simulink model "SingleTrackCANoe"  (R2021b)
settings: Solver=ode1  StartTime=0  StopTime=2  FixedStep=1.0000000000000000e-003  RelTol=1e-3
InitFcn:
  | sampleTime = str2double(get_param(bdroot, 'FixedStep'));
undefined symbols (not defined in the file or in its folder): AccPedalPos, BrakePedalPos, BrakeSwitch, DiscIntNeverNeededParam, DYNA4, EngSpd, IgnitionSwitch, InitialGear, InitialSpeed, IntendedEngTrq, LeftIndicator, MainBrakePress, MaxGear, MDL, MinGear, RefAcc, RefLane, RefLatPos, RefPath, RefPathCurv, RefSpd, RefSpdPreview, RefSpdRetrospect, RightIndicator, SteeringWheelAng, SteeringWheelTrq, UserDefinedRefValue, vm_const
libraries: UtilitiesLibrary x62, simulink x18, WheelSystemModules x14, LongitudinalControllerModules x13, LateralControllerModules x7, AnimationBusselectorModules x5, EnvironmentModules x5, BasicEngineControlModules x5, MiscellaneousControlModules x5, Animation3Modules x4, AuxiliariesModules x4, ReducedTireModules x4
(part 32 of 34)

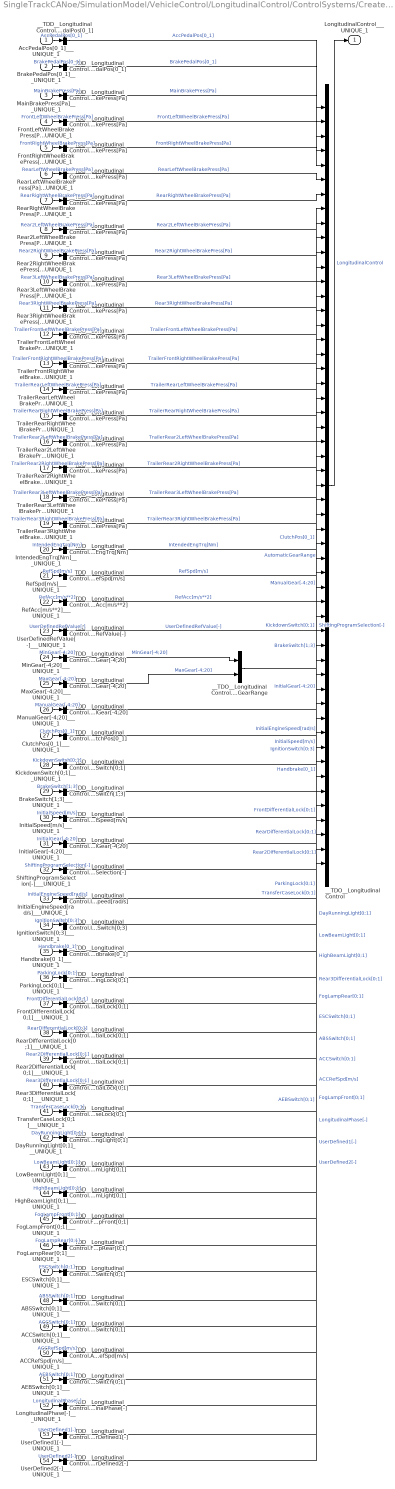
== system SingleTrackCANoe/SimulationModel/VehicleControl/LongitudinalControl/ControlSystems/CreateOutputBus/LongitudinalControlOutput ==
  AccPedalPos[0_1]___UNIQUE_1 : Inport  Description=|  PortDimensions=[1]
      | <name>AccPedalPos[0_1]</name>
      | <comment>Accelerator pedal position</comment>
  BrakePedalPos[0_1]___UNIQUE_1 : Inport  Description=|  Port=2  PortDimensions=[1]
      | <name>BrakePedalPos[0_1]</name>
      | <comment>Brake pedal position</comment>
  MainBrakePress[Pa]___UNIQUE_1 : Inport  Description=|  Port=3  PortDimensions=[1]
      | <name>MainBrakePress[Pa]</name>
      | <comment>Main brake pressure</comment>
  FrontLeftWheelBrakePress[Pa]___UNIQUE_1 : Inport  Description=|  Port=4  PortDimensions=[1]
      | <name>FrontLeftWheelBrakePress[Pa]</name>
      | <comment>Front axle left wheel brake pressure</comment>
  FrontRightWheelBrakePress[Pa]___UNIQUE_1 : Inport  Description=|  Port=5  PortDimensions=[1]
      | <name>FrontRightWheelBrakePress[Pa]</name>
      | <comment>Front axle right wheel brake pressure</comment>
  RearLeftWheelBrakePress[Pa]___UNIQUE_1 : Inport  Description=|  Port=6  PortDimensions=[1]
      | <name>RearLeftWheelBrakePress[Pa]</name>
      | <comment>Rear axle left wheel brake pressure</comment>
  RearRightWheelBrakePress[Pa]___UNIQUE_1 : Inport  Description=|  Port=7  PortDimensions=[1]
      | <name>RearRightWheelBrakePress[Pa]</name>
      | <comment>Rear axle right wheel brake pressure</comment>
  Rear2LeftWheelBrakePress[Pa]___UNIQUE_1 : Inport  Description=|  Port=8  PortDimensions=[1]
      | <name>Rear2LeftWheelBrakePress[Pa]</name>
      | <comment>Second rear axle left wheel brake pressure</comment>
  Rear2RightWheelBrakePress[Pa]___UNIQUE_1 : Inport  Description=|  Port=9  PortDimensions=[1]
      | <name>Rear2RightWheelBrakePress[Pa]</name>
      | <comment>Second rear axle right wheel brake pressure</comment>
  Rear3LeftWheelBrakePress[Pa]___UNIQUE_1 : Inport  Description=|  Port=10  PortDimensions=[1]
      | <name>Rear3LeftWheelBrakePress[Pa]</name>
      | <comment>Third rear axle left wheel brake pressure</comment>
  Rear3RightWheelBrakePress[Pa]___UNIQUE_1 : Inport  Description=|  Port=11  PortDimensions=[1]
      | <name>Rear3RightWheelBrakePress[Pa]</name>
      | <comment>Third rear axle right wheel brake pressure</comment>
  TrailerFrontLeftWheelBrakePress[Pa]___UNIQUE_1 : Inport  Description=|  Port=12  PortDimensions=[1]
      | <name>TrailerFrontLeftWheelBrakePress[Pa]</name>
      | <comment>Trailer front axle left wheel brake pressure</comment>
  TrailerFrontRightWheelBrakePress[Pa]___UNIQUE_1 : Inport  Description=|  Port=13  PortDimensions=[1]
      | <name>TrailerFrontRightWheelBrakePress[Pa]</name>
      | <comment>Trailer front axle right wheel brake pressure</comment>
  TrailerRearLeftWheelBrakePress[Pa]___UNIQUE_1 : Inport  Description=|  Port=14  PortDimensions=[1]
      | <name>TrailerRearLeftWheelBrakePress[Pa]</name>
      | <comment>Trailer rear axle left wheel brake pressure</comment>
  TrailerRearRightWheelBrakePress[Pa]___UNIQUE_1 : Inport  Description=|  Port=15  PortDimensions=[1]
      | <name>TrailerRearRightWheelBrakePress[Pa]</name>
      | <comment>Trailer rear axle right wheel brake pressure</comment>
  TrailerRear2LeftWheelBrakePress[Pa]___UNIQUE_1 : Inport  Description=|  Port=16  PortDimensions=[1]
      | <name>TrailerRear2LeftWheelBrakePress[Pa]</name>
      | <comment>Trailer second rear axle left wheel brake pressure</comment>
  TrailerRear2RightWheelBrakePress[Pa]___UNIQUE_1 : Inport  Description=|  Port=17  PortDimensions=[1]
      | <name>TrailerRear2RightWheelBrakePress[Pa]</name>
      | <comment>Trailer second rear axle right wheel brake pressure</comment>
  TrailerRear3LeftWheelBrakePress[Pa]___UNIQUE_1 : Inport  Description=|  Port=18  PortDimensions=[1]
      | <name>TrailerRear3LeftWheelBrakePress[Pa]</name>
      | <comment>Trailer third rear axle left wheel brake pressure</comment>
  TrailerRear3RightWheelBrakePress[Pa]___UNIQUE_1 : Inport  Description=|  Port=19  PortDimensions=[1]
      | <name>TrailerRear3RightWheelBrakePress[Pa]</name>
      | <comment>Trailer third rear axle right wheel brake pressure</comment>
  IntendedEngTrq[Nm]___UNIQUE_1 : Inport  Description=|  Port=20  PortDimensions=[1]
      | <name>IntendedEngTrq[Nm]</name>
      | <comment>Intended engine torque</comment>
  RefSpd[m/s]___UNIQUE_1 : Inport  Description=|  Port=21  PortDimensions=[1]
      | <name>RefSpd[m/s]</name>
      | <comment>Vehicle reference speed</comment>
  RefAcc[m/s**2]___UNIQUE_1 : Inport  Description=|  Port=22  PortDimensions=[1]
      | <name>RefAcc[m/s**2]</name>
      | <comment></comment>
  UserDefinedRefValue[-]___UNIQUE_1 : Inport  Description=|  Port=23  PortDimensions=[1]
      | <name>UserDefinedRefValue[-]</name>
      | <comment>User-defined reference value</comment>
  MinGear[-4;20]___UNIQUE_1 : Inport  Description=|  Port=24  PortDimensions=[1]
      | <name>MinGear[-4;20]</name>
      | <comment>Minimum gear</comment>
  MaxGear[-4;20]___UNIQUE_1 : Inport  Description=|  Port=25  PortDimensions=[1]
      | <name>MaxGear[-4;20]</name>
      | <comment>Maximum gear</comment>
  ManualGear[-4;20]___UNIQUE_1 : Inport  Description=|  Port=26  PortDimensions=[1]
      | <name>ManualGear[-4;20]</name>
      | <comment>Gear number for manual transmission</comment>
  ClutchPos[0_1]___UNIQUE_1 : Inport  Description=|  Port=27  PortDimensions=[1]
      | <name>ClutchPos[0_1]</name>
      | <comment>Clutch position</comment>
  KickdownSwitch[0;1]___UNIQUE_1 : Inport  Description=|  Port=28  PortDimensions=[1]
      | <name>KickdownSwitch[0;1]</name>
      | <comment>Kickdown switch</comment>
  BrakeSwitch[1;3]___UNIQUE_1 : Inport  Description=|  Port=29  PortDimensions=[1]
      | <name>BrakeSwitch[1;3]</name>
      | <comment>Logical switch for brake system control, 1: Main and wheel brake pressures are calculated from the supplied brake pedal position, 2: Wheel brake pressures are calculated from the supplied main brake pressure, 3: Wheel brake pressures are supplied directly </comment>
  InitialSpeed[m/s]___UNIQUE_1 : Inport  Description=|  Port=30  PortDimensions=[1]
      | <name>InitialSpeed[m/s]</name>
      | <comment>Initial vehicle speed</comment>
  InitialGear[-4;20]___UNIQUE_1 : Inport  Description=|  Port=31  PortDimensions=[1]
      | <name>InitialGear[-4;20]</name>
      | <comment>Initial gear</comment>
  ShiftingProgramSelection[-]___UNIQUE_1 : Inport  Description=|  Port=32  PortDimensions=[1]
      | <name>ShiftingProgramSelection[-]</name>
      | <comment>Selection of shifting program number</comment>
  InitialEngineSpeed[rad/s]___UNIQUE_1 : Inport  Description=|  Port=33  PortDimensions=[1]
      | <name>InitialEngineSpeed[rad/s]</name>
      | <comment>Initial engine speed</comment>
  IgnitionSwitch[0;3]___UNIQUE_1 : Inport  Description=|  Port=34  PortDimensions=[1]
      | <name>IgnitionSwitch[0;3]</name>
      | <comment>Ignition switch, 0: Ignition is off,  1: Only limited electric power supply, e.g for the radio, is available, 2: Normal operation mode: Full electric power supply is available, 3: Starter is activated</comment>
  Handbrake[0_1]___UNIQUE_1 : Inport  Description=|  Port=35  PortDimensions=[1]
      | <name>Handbrake[0_1]</name>
      | <comment>Handbrake position</comment>
  ParkingLock[0;1]___UNIQUE_1 : Inport  Description=|  Port=36  PortDimensions=[1]
      | <name>ParkingLock[0;1]</name>
      | <comment>Parking lock state</comment>
  FrontDifferentialLock[0;1]___UNIQUE_1 : Inport  Description=|  Port=37  PortDimensions=[1]
      | <name>FrontDifferentialLock[0;1]</name>
      | <comment>Front differential lock state</comment>
  RearDifferentialLock[0;1]___UNIQUE_1 : Inport  Description=|  Port=38  PortDimensions=[1]
      | <name>RearDifferentialLock[0;1]</name>
      | <comment>Rear differential lock state</comment>
  Rear2DifferentialLock[0;1]___UNIQUE_1 : Inport  Description=|  Port=39  PortDimensions=[1]
      | <name>Rear2DifferentialLock[0;1]</name>
      | <comment>Second rear differential lock state</comment>
  Rear3DifferentialLock[0;1]___UNIQUE_1 : Inport  Description=|  Port=40  PortDimensions=[1]
      | <name>Rear3DifferentialLock[0;1]</name>
      | <comment>Third rear differential lock state</comment>
  TransferCaseLock[0;1]___UNIQUE_1 : Inport  Description=|  Port=41  PortDimensions=[1]
      | <name>TransferCaseLock[0;1]</name>
      | <comment>Transfer case lock state</comment>
  DayRunningLight[0;1]___UNIQUE_1 : Inport  Description=|  Port=42  PortDimensions=[1]
      | <name>DayRunningLight[0;1]</name>
      | <comment></comment>
  LowBeamLight[0;1]___UNIQUE_1 : Inport  Description=|  Port=43  PortDimensions=[1]
      | <name>LowBeamLight[0;1]</name>
      | <comment></comment>
  HighBeamLight[0;1]___UNIQUE_1 : Inport  Description=|  Port=44  PortDimensions=[1]
      | <name>HighBeamLight[0;1]</name>
      | <comment></comment>
  FogLampFront[0;1]___UNIQUE_1 : Inport  Description=|  Port=45  PortDimensions=[1]
      | <name>FogLampFront[0;1]</name>
      | <comment></comment>
  FogLampRear[0;1]___UNIQUE_1 : Inport  Description=|  Port=46  PortDimensions=[1]
      | <name>FogLampRear[0;1]</name>
      | <comment></comment>
  ESCSwitch[0;1]___UNIQUE_1 : Inport  Description=|  Port=47  PortDimensions=[1]
      | <name>ESCSwitch[0;1]</name>
      | <comment>ESC activation switch</comment>
  ABSSwitch[0;1]___UNIQUE_1 : Inport  Description=|  Port=48  PortDimensions=[1]
      | <name>ABSSwitch[0;1]</name>
      | <comment>ABS activation switch</comment>
  ACCSwitch[0;1]___UNIQUE_1 : Inport  Description=|  Port=49  PortDimensions=[1]
      | <name>ACCSwitch[0;1]</name>
      | <comment></comment>
  ACCRefSpd[m/s]___UNIQUE_1 : Inport  Description=|  Port=50  PortDimensions=[1]
      | <name>ACCRefSpd[m/s]</name>
      | <comment></comment>
  AEBSwitch[0;1]___UNIQUE_1 : Inport  Description=|  Port=51  PortDimensions=[1]
      | <name>AEBSwitch[0;1]</name>
      | <comment></comment>
  LongitudinalPhase[-]___UNIQUE_1 : Inport  Description=|  Port=52  PortDimensions=[1]
      | <name>LongitudinalPhase[-]</name>
      | <comment>Longitudinal phase number</comment>
  UserDefined1[-]___UNIQUE_1 : Inport  Description=|  Port=53  PortDimensions=[1]
      | <name>UserDefined.UserDefined1[-]</name>
      | <comment>User-defined additional input 1 (can be edited by the user)</comment>
  UserDefined2[-]___UNIQUE_1 : Inport  Description=|  Port=54  PortDimensions=[1]
      | <name>UserDefined.UserDefined2[-]</name>
      | <comment>User-defined additional input 2 (can be edited by the user)</comment>
  __TDD__LongitudinalControl.ABSSwitch[0;1] : Demux  Outputs=[1]
  __TDD__LongitudinalControl.ACCRefSpd[m/s] : Demux  Outputs=[1]
  __TDD__LongitudinalControl.ACCSwitch[0;1] : Demux  Outputs=[1]
  __TDD__LongitudinalControl.AEBSwitch[0;1] : Demux  Outputs=[1]
  __TDD__LongitudinalControl.AccPedalPos[0_1] : Demux  Outputs=[1]
  __TDD__LongitudinalControl.AutomaticGearRange.MaxGear[-4;20] : Demux  Outputs=[1]
  __TDD__LongitudinalControl.AutomaticGearRange.MinGear[-4;20] : Demux  Outputs=[1]
  __TDD__LongitudinalControl.BrakePedalPos[0_1] : Demux  Outputs=[1]
  __TDD__LongitudinalControl.BrakeSwitch[1;3] : Demux  Outputs=[1]
  __TDD__LongitudinalControl.ClutchPos[0_1] : Demux  Outputs=[1]
  __TDD__LongitudinalControl.DayRunningLight[0;1] : Demux  Outputs=[1]
  __TDD__LongitudinalControl.ESCSwitch[0;1] : Demux  Outputs=[1]
  __TDD__LongitudinalControl.FogLampFront[0;1] : Demux  Outputs=[1]
  __TDD__LongitudinalControl.FogLampRear[0;1] : Demux  Outputs=[1]
  __TDD__LongitudinalControl.FrontDifferentialLock[0;1] : Demux  Outputs=[1]
  __TDD__LongitudinalControl.FrontLeftWheelBrakePress[Pa] : Demux  Outputs=[1]
  __TDD__LongitudinalControl.FrontRightWheelBrakePress[Pa] : Demux  Outputs=[1]
  __TDD__LongitudinalControl.Handbrake[0_1] : Demux  Outputs=[1]
  __TDD__LongitudinalControl.HighBeamLight[0;1] : Demux  Outputs=[1]
  __TDD__LongitudinalControl.IgnitionSwitch[0;3] : Demux  Outputs=[1]
  __TDD__LongitudinalControl.InitialEngineSpeed[rad/s] : Demux  Outputs=[1]
  __TDD__LongitudinalControl.InitialGear[-4;20] : Demux  Outputs=[1]
  __TDD__LongitudinalControl.InitialSpeed[m/s] : Demux  Outputs=[1]
  __TDD__LongitudinalControl.IntendedEngTrq[Nm] : Demux  Outputs=[1]
  __TDD__LongitudinalControl.KickdownSwitch[0;1] : Demux  Outputs=[1]
  __TDD__LongitudinalControl.LongitudinalPhase[-] : Demux  Outputs=[1]
  __TDD__LongitudinalControl.LowBeamLight[0;1] : Demux  Outputs=[1]
  __TDD__LongitudinalControl.MainBrakePress[Pa] : Demux  Outputs=[1]
  __TDD__LongitudinalControl.ManualGear[-4;20] : Demux  Outputs=[1]
  __TDD__LongitudinalControl.ParkingLock[0;1] : Demux  Outputs=[1]
  __TDD__LongitudinalControl.Rear2DifferentialLock[0;1] : Demux  Outputs=[1]
  __TDD__LongitudinalControl.Rear2LeftWheelBrakePress[Pa] : Demux  Outputs=[1]
  __TDD__LongitudinalControl.Rear2RightWheelBrakePress[Pa] : Demux  Outputs=[1]
  __TDD__LongitudinalControl.Rear3DifferentialLock[0;1] : Demux  Outputs=[1]
  __TDD__LongitudinalControl.Rear3LeftWheelBrakePress[Pa] : Demux  Outputs=[1]
  __TDD__LongitudinalControl.Rear3RightWheelBrakePress[Pa] : Demux  Outputs=[1]
  __TDD__LongitudinalControl.RearDifferentialLock[0;1] : Demux  Outputs=[1]
  __TDD__LongitudinalControl.RearLeftWheelBrakePress[Pa] : Demux  Outputs=[1]
  __TDD__LongitudinalControl.RearRightWheelBrakePress[Pa] : Demux  Outputs=[1]
  __TDD__LongitudinalControl.RefAcc[m/s**2] : Demux  Outputs=[1]
  __TDD__LongitudinalControl.RefSpd[m/s] : Demux  Outputs=[1]
  __TDD__LongitudinalControl.ShiftingProgramSelection[-] : Demux  Outputs=[1]
  __TDD__LongitudinalControl.TrailerFrontLeftWheelBrakePress[Pa] : Demux  Outputs=[1]
  __TDD__LongitudinalControl.TrailerFrontRightWheelBrakePress[Pa] : Demux  Outputs=[1]
  __TDD__LongitudinalControl.TrailerRear2LeftWheelBrakePress[Pa] : Demux  Outputs=[1]
  __TDD__LongitudinalControl.TrailerRear2RightWheelBrakePress[Pa] : Demux  Outputs=[1]
  __TDD__LongitudinalControl.TrailerRear3LeftWheelBrakePress[Pa] : Demux  Outputs=[1]
  __TDD__LongitudinalControl.TrailerRear3RightWheelBrakePress[Pa] : Demux  Outputs=[1]
  __TDD__LongitudinalControl.TrailerRearLeftWheelBrakePress[Pa] : Demux  Outputs=[1]
  __TDD__LongitudinalControl.TrailerRearRightWheelBrakePress[Pa] : Demux  Outputs=[1]
  __TDD__LongitudinalControl.TransferCaseLock[0;1] : Demux  Outputs=[1]
  __TDD__LongitudinalControl.UserDefined1[-] : Demux  Outputs=[1]
  __TDD__LongitudinalControl.UserDefined2[-] : Demux  Outputs=[1]
  __TDD__LongitudinalControl.UserDefinedRefValue[-] : Demux  Outputs=[1]
  __TDO__LongitudinalControl : BusCreator  Inputs=53
  __TDO__LongitudinalControl.AutomaticGearRange : BusCreator  Inputs=2
  LongitudinalControl___UNIQUE_1 : Outport  Description=|  PortDimensions=[54]  VectorParamsAs1DForOutWhenUnconnected=off
      | <name>AccPedalPos[0_1]</name>
      | <comment>Accelerator pedal position</comment>
  wires:
  AccPedalPos[0_1]___UNIQUE_1/1 -> __TDD__LongitudinalControl.AccPedalPos[0_1]/1  "AccPedalPos[0_1]"
  __TDD__LongitudinalControl.AccPedalPos[0_1]/1 -> __TDO__LongitudinalControl/1  "AccPedalPos[0_1]"
  BrakePedalPos[0_1]___UNIQUE_1/1 -> __TDD__LongitudinalControl.BrakePedalPos[0_1]/1  "BrakePedalPos[0_1]"
  __TDD__LongitudinalControl.BrakePedalPos[0_1]/1 -> __TDO__LongitudinalControl/2  "BrakePedalPos[0_1]"
  MainBrakePress[Pa]___UNIQUE_1/1 -> __TDD__LongitudinalControl.MainBrakePress[Pa]/1  "MainBrakePress[Pa]"
  __TDD__LongitudinalControl.MainBrakePress[Pa]/1 -> __TDO__LongitudinalControl/3  "MainBrakePress[Pa]"
  FrontLeftWheelBrakePress[Pa]___UNIQUE_1/1 -> __TDD__LongitudinalControl.FrontLeftWheelBrakePress[Pa]/1  "FrontLeftWheelBrakePress[Pa]"
  __TDD__LongitudinalControl.FrontLeftWheelBrakePress[Pa]/1 -> __TDO__LongitudinalControl/4  "FrontLeftWheelBrakePress[Pa]"
  FrontRightWheelBrakePress[Pa]___UNIQUE_1/1 -> __TDD__LongitudinalControl.FrontRightWheelBrakePress[Pa]/1  "FrontRightWheelBrakePress[Pa]"
  __TDD__LongitudinalControl.FrontRightWheelBrakePress[Pa]/1 -> __TDO__LongitudinalControl/5  "FrontRightWheelBrakePress[Pa]"
  RearLeftWheelBrakePress[Pa]___UNIQUE_1/1 -> __TDD__LongitudinalControl.RearLeftWheelBrakePress[Pa]/1  "RearLeftWheelBrakePress[Pa]"
  __TDD__LongitudinalControl.RearLeftWheelBrakePress[Pa]/1 -> __TDO__LongitudinalControl/6  "RearLeftWheelBrakePress[Pa]"
  RearRightWheelBrakePress[Pa]___UNIQUE_1/1 -> __TDD__LongitudinalControl.RearRightWheelBrakePress[Pa]/1  "RearRightWheelBrakePress[Pa]"
  __TDD__LongitudinalControl.RearRightWheelBrakePress[Pa]/1 -> __TDO__LongitudinalControl/7  "RearRightWheelBrakePress[Pa]"
  Rear2LeftWheelBrakePress[Pa]___UNIQUE_1/1 -> __TDD__LongitudinalControl.Rear2LeftWheelBrakePress[Pa]/1  "Rear2LeftWheelBrakePress[Pa]"
  __TDD__LongitudinalControl.Rear2LeftWheelBrakePress[Pa]/1 -> __TDO__LongitudinalControl/8  "Rear2LeftWheelBrakePress[Pa]"
  Rear2RightWheelBrakePress[Pa]___UNIQUE_1/1 -> __TDD__LongitudinalControl.Rear2RightWheelBrakePress[Pa]/1  "Rear2RightWheelBrakePress[Pa]"
  __TDD__LongitudinalControl.Rear2RightWheelBrakePress[Pa]/1 -> __TDO__LongitudinalControl/9  "Rear2RightWheelBrakePress[Pa]"
  Rear3LeftWheelBrakePress[Pa]___UNIQUE_1/1 -> __TDD__LongitudinalControl.Rear3LeftWheelBrakePress[Pa]/1  "Rear3LeftWheelBrakePress[Pa]"
  __TDD__LongitudinalControl.Rear3LeftWheelBrakePress[Pa]/1 -> __TDO__LongitudinalControl/10  "Rear3LeftWheelBrakePress[Pa]"
  Rear3RightWheelBrakePress[Pa]___UNIQUE_1/1 -> __TDD__LongitudinalControl.Rear3RightWheelBrakePress[Pa]/1  "Rear3RightWheelBrakePress[Pa]"
  __TDD__LongitudinalControl.Rear3RightWheelBrakePress[Pa]/1 -> __TDO__LongitudinalControl/11  "Rear3RightWheelBrakePress[Pa]"
  TrailerFrontLeftWheelBrakePress[Pa]___UNIQUE_1/1 -> __TDD__LongitudinalControl.TrailerFrontLeftWheelBrakePress[Pa]/1  "TrailerFrontLeftWheelBrakePress[Pa]"
  __TDD__LongitudinalControl.TrailerFrontLeftWheelBrakePress[Pa]/1 -> __TDO__LongitudinalControl/12  "TrailerFrontLeftWheelBrakePress[Pa]"
  TrailerFrontRightWheelBrakePress[Pa]___UNIQUE_1/1 -> __TDD__LongitudinalControl.TrailerFrontRightWheelBrakePress[Pa]/1  "TrailerFrontRightWheelBrakePress[Pa]"
  __TDD__LongitudinalControl.TrailerFrontRightWheelBrakePress[Pa]/1 -> __TDO__LongitudinalControl/13  "TrailerFrontRightWheelBrakePress[Pa]"
  TrailerRearLeftWheelBrakePress[Pa]___UNIQUE_1/1 -> __TDD__LongitudinalControl.TrailerRearLeftWheelBrakePress[Pa]/1  "TrailerRearLeftWheelBrakePress[Pa]"
  __TDD__LongitudinalControl.TrailerRearLeftWheelBrakePress[Pa]/1 -> __TDO__LongitudinalControl/14  "TrailerRearLeftWheelBrakePress[Pa]"
  TrailerRearRightWheelBrakePress[Pa]___UNIQUE_1/1 -> __TDD__LongitudinalControl.TrailerRearRightWheelBrakePress[Pa]/1  "TrailerRearRightWheelBrakePress[Pa]"
  __TDD__LongitudinalControl.TrailerRearRightWheelBrakePress[Pa]/1 -> __TDO__LongitudinalControl/15  "TrailerRearRightWheelBrakePress[Pa]"
  TrailerRear2LeftWheelBrakePress[Pa]___UNIQUE_1/1 -> __TDD__LongitudinalControl.TrailerRear2LeftWheelBrakePress[Pa]/1  "TrailerRear2LeftWheelBrakePress[Pa]"
  __TDD__LongitudinalControl.TrailerRear2LeftWheelBrakePress[Pa]/1 -> __TDO__LongitudinalControl/16  "TrailerRear2LeftWheelBrakePress[Pa]"
  TrailerRear2RightWheelBrakePress[Pa]___UNIQUE_1/1 -> __TDD__LongitudinalControl.TrailerRear2RightWheelBrakePress[Pa]/1  "TrailerRear2RightWheelBrakePress[Pa]"
  __TDD__LongitudinalControl.TrailerRear2RightWheelBrakePress[Pa]/1 -> __TDO__LongitudinalControl/17  "TrailerRear2RightWheelBrakePress[Pa]"
  TrailerRear3LeftWheelBrakePress[Pa]___UNIQUE_1/1 -> __TDD__LongitudinalControl.TrailerRear3LeftWheelBrakePress[Pa]/1  "TrailerRear3LeftWheelBrakePress[Pa]"
  __TDD__LongitudinalControl.TrailerRear3LeftWheelBrakePress[Pa]/1 -> __TDO__LongitudinalControl/18  "TrailerRear3LeftWheelBrakePress[Pa]"
  TrailerRear3RightWheelBrakePress[Pa]___UNIQUE_1/1 -> __TDD__LongitudinalControl.TrailerRear3RightWheelBrakePress[Pa]/1  "TrailerRear3RightWheelBrakePress[Pa]"
  __TDD__LongitudinalControl.TrailerRear3RightWheelBrakePress[Pa]/1 -> __TDO__LongitudinalControl/19  "TrailerRear3RightWheelBrakePress[Pa]"
  IntendedEngTrq[Nm]___UNIQUE_1/1 -> __TDD__LongitudinalControl.IntendedEngTrq[Nm]/1  "IntendedEngTrq[Nm]"
  __TDD__LongitudinalControl.IntendedEngTrq[Nm]/1 -> __TDO__LongitudinalControl/20  "IntendedEngTrq[Nm]"
  RefSpd[m/s]___UNIQUE_1/1 -> __TDD__LongitudinalControl.RefSpd[m/s]/1  "RefSpd[m/s]"
  __TDD__LongitudinalControl.RefSpd[m/s]/1 -> __TDO__LongitudinalControl/21  "RefSpd[m/s]"
  RefAcc[m/s**2]___UNIQUE_1/1 -> __TDD__LongitudinalControl.RefAcc[m/s**2]/1  "RefAcc[m/s**2]"
  __TDD__LongitudinalControl.RefAcc[m/s**2]/1 -> __TDO__LongitudinalControl/22  "RefAcc[m/s**2]"
  UserDefinedRefValue[-]___UNIQUE_1/1 -> __TDD__LongitudinalControl.UserDefinedRefValue[-]/1  "UserDefinedRefValue[-]"
  __TDD__LongitudinalControl.UserDefinedRefValue[-]/1 -> __TDO__LongitudinalControl/23  "UserDefinedRefValue[-]"
  MinGear[-4;20]___UNIQUE_1/1 -> __TDD__LongitudinalControl.AutomaticGearRange.MinGear[-4;20]/1  "MinGear[-4;20]"
  __TDD__LongitudinalControl.AutomaticGearRange.MinGear[-4;20]/1 -> __TDO__LongitudinalControl.AutomaticGearRange/1  "MinGear[-4;20]"
  __TDO__LongitudinalControl.AutomaticGearRange/1 -> __TDO__LongitudinalControl/24  "AutomaticGearRange"
  MaxGear[-4;20]___UNIQUE_1/1 -> __TDD__LongitudinalControl.AutomaticGearRange.MaxGear[-4;20]/1  "MaxGear[-4;20]"
  __TDD__LongitudinalControl.AutomaticGearRange.MaxGear[-4;20]/1 -> __TDO__LongitudinalControl.AutomaticGearRange/2  "MaxGear[-4;20]"
  ManualGear[-4;20]___UNIQUE_1/1 -> __TDD__LongitudinalControl.ManualGear[-4;20]/1  "ManualGear[-4;20]"
  __TDD__LongitudinalControl.ManualGear[-4;20]/1 -> __TDO__LongitudinalControl/25  "ManualGear[-4;20]"
  ClutchPos[0_1]___UNIQUE_1/1 -> __TDD__LongitudinalControl.ClutchPos[0_1]/1  "ClutchPos[0_1]"
  __TDD__LongitudinalControl.ClutchPos[0_1]/1 -> __TDO__LongitudinalControl/26  "ClutchPos[0_1]"
  KickdownSwitch[0;1]___UNIQUE_1/1 -> __TDD__LongitudinalControl.KickdownSwitch[0;1]/1  "KickdownSwitch[0;1]"
  __TDD__LongitudinalControl.KickdownSwitch[0;1]/1 -> __TDO__LongitudinalControl/27  "KickdownSwitch[0;1]"
  BrakeSwitch[1;3]___UNIQUE_1/1 -> __TDD__LongitudinalControl.BrakeSwitch[1;3]/1  "BrakeSwitch[1;3]"
  __TDD__LongitudinalControl.BrakeSwitch[1;3]/1 -> __TDO__LongitudinalControl/28  "BrakeSwitch[1;3]"
  InitialSpeed[m/s]___UNIQUE_1/1 -> __TDD__LongitudinalControl.InitialSpeed[m/s]/1  "InitialSpeed[m/s]"
  __TDD__LongitudinalControl.InitialSpeed[m/s]/1 -> __TDO__LongitudinalControl/29  "InitialSpeed[m/s]"
  InitialGear[-4;20]___UNIQUE_1/1 -> __TDD__LongitudinalControl.InitialGear[-4;20]/1  "InitialGear[-4;20]"
  __TDD__LongitudinalControl.InitialGear[-4;20]/1 -> __TDO__LongitudinalControl/30  "InitialGear[-4;20]"
  ShiftingProgramSelection[-]___UNIQUE_1/1 -> __TDD__LongitudinalControl.ShiftingProgramSelection[-]/1  "ShiftingProgramSelection[-]"
  __TDD__LongitudinalControl.ShiftingProgramSelection[-]/1 -> __TDO__LongitudinalControl/31  "ShiftingProgramSelection[-]"
  InitialEngineSpeed[rad/s]___UNIQUE_1/1 -> __TDD__LongitudinalControl.InitialEngineSpeed[rad/s]/1  "InitialEngineSpeed[rad/s]"
  __TDD__LongitudinalControl.InitialEngineSpeed[rad/s]/1 -> __TDO__LongitudinalControl/32  "InitialEngineSpeed[rad/s]"
  IgnitionSwitch[0;3]___UNIQUE_1/1 -> __TDD__LongitudinalControl.IgnitionSwitch[0;3]/1  "IgnitionSwitch[0;3]"
  __TDD__LongitudinalControl.IgnitionSwitch[0;3]/1 -> __TDO__LongitudinalControl/33  "IgnitionSwitch[0;3]"
  Handbrake[0_1]___UNIQUE_1/1 -> __TDD__LongitudinalControl.Handbrake[0_1]/1  "Handbrake[0_1]"
  __TDD__LongitudinalControl.Handbrake[0_1]/1 -> __TDO__LongitudinalControl/34  "Handbrake[0_1]"
  ParkingLock[0;1]___UNIQUE_1/1 -> __TDD__LongitudinalControl.ParkingLock[0;1]/1  "ParkingLock[0;1]"
  __TDD__LongitudinalControl.ParkingLock[0;1]/1 -> __TDO__LongitudinalControl/35  "ParkingLock[0;1]"
  FrontDifferentialLock[0;1]___UNIQUE_1/1 -> __TDD__LongitudinalControl.FrontDifferentialLock[0;1]/1  "FrontDifferentialLock[0;1]"
  __TDD__LongitudinalControl.FrontDifferentialLock[0;1]/1 -> __TDO__LongitudinalControl/36  "FrontDifferentialLock[0;1]"
  RearDifferentialLock[0;1]___UNIQUE_1/1 -> __TDD__LongitudinalControl.RearDifferentialLock[0;1]/1  "RearDifferentialLock[0;1]"
  __TDD__LongitudinalControl.RearDifferentialLock[0;1]/1 -> __TDO__LongitudinalControl/37  "RearDifferentialLock[0;1]"
  Rear2DifferentialLock[0;1]___UNIQUE_1/1 -> __TDD__LongitudinalControl.Rear2DifferentialLock[0;1]/1  "Rear2DifferentialLock[0;1]"
  __TDD__LongitudinalControl.Rear2DifferentialLock[0;1]/1 -> __TDO__LongitudinalControl/38  "Rear2DifferentialLock[0;1]"
  Rear3DifferentialLock[0;1]___UNIQUE_1/1 -> __TDD__LongitudinalControl.Rear3DifferentialLock[0;1]/1  "Rear3DifferentialLock[0;1]"
  __TDD__LongitudinalControl.Rear3DifferentialLock[0;1]/1 -> __TDO__LongitudinalControl/39  "Rear3DifferentialLock[0;1]"
  TransferCaseLock[0;1]___UNIQUE_1/1 -> __TDD__LongitudinalControl.TransferCaseLock[0;1]/1  "TransferCaseLock[0;1]"
  __TDD__LongitudinalControl.TransferCaseLock[0;1]/1 -> __TDO__LongitudinalControl/40  "TransferCaseLock[0;1]"
  DayRunningLight[0;1]___UNIQUE_1/1 -> __TDD__LongitudinalControl.DayRunningLight[0;1]/1  "DayRunningLight[0;1]"
  __TDD__LongitudinalControl.DayRunningLight[0;1]/1 -> __TDO__LongitudinalControl/41  "DayRunningLight[0;1]"
  LowBeamLight[0;1]___UNIQUE_1/1 -> __TDD__LongitudinalControl.LowBeamLight[0;1]/1  "LowBeamLight[0;1]"
  __TDD__LongitudinalControl.LowBeamLight[0;1]/1 -> __TDO__LongitudinalControl/42  "LowBeamLight[0;1]"
  HighBeamLight[0;1]___UNIQUE_1/1 -> __TDD__LongitudinalControl.HighBeamLight[0;1]/1  "HighBeamLight[0;1]"
  __TDD__LongitudinalControl.HighBeamLight[0;1]/1 -> __TDO__LongitudinalControl/43  "HighBeamLight[0;1]"
  FogLampFront[0;1]___UNIQUE_1/1 -> __TDD__LongitudinalControl.FogLampFront[0;1]/1  "FogLampFront[0;1]"
  __TDD__LongitudinalControl.FogLampFront[0;1]/1 -> __TDO__LongitudinalControl/44  "FogLampFront[0;1]"
  FogLampRear[0;1]___UNIQUE_1/1 -> __TDD__LongitudinalControl.FogLampRear[0;1]/1  "FogLampRear[0;1]"
  __TDD__LongitudinalControl.FogLampRear[0;1]/1 -> __TDO__LongitudinalControl/45  "FogLampRear[0;1]"
  ESCSwitch[0;1]___UNIQUE_1/1 -> __TDD__LongitudinalControl.ESCSwitch[0;1]/1  "ESCSwitch[0;1]"
  __TDD__LongitudinalControl.ESCSwitch[0;1]/1 -> __TDO__LongitudinalControl/46  "ESCSwitch[0;1]"
  ABSSwitch[0;1]___UNIQUE_1/1 -> __TDD__LongitudinalControl.ABSSwitch[0;1]/1  "ABSSwitch[0;1]"
  __TDD__LongitudinalControl.ABSSwitch[0;1]/1 -> __TDO__LongitudinalControl/47  "ABSSwitch[0;1]"
  ACCSwitch[0;1]___UNIQUE_1/1 -> __TDD__LongitudinalControl.ACCSwitch[0;1]/1  "ACCSwitch[0;1]"
  __TDD__LongitudinalControl.ACCSwitch[0;1]/1 -> __TDO__LongitudinalControl/48  "ACCSwitch[0;1]"
  ACCRefSpd[m/s]___UNIQUE_1/1 -> __TDD__LongitudinalControl.ACCRefSpd[m/s]/1  "ACCRefSpd[m/s]"
  __TDD__LongitudinalControl.ACCRefSpd[m/s]/1 -> __TDO__LongitudinalControl/49  "ACCRefSpd[m/s]"
  AEBSwitch[0;1]___UNIQUE_1/1 -> __TDD__LongitudinalControl.AEBSwitch[0;1]/1  "AEBSwitch[0;1]"
  __TDD__LongitudinalControl.AEBSwitch[0;1]/1 -> __TDO__LongitudinalControl/50  "AEBSwitch[0;1]"
  LongitudinalPhase[-]___UNIQUE_1/1 -> __TDD__LongitudinalControl.LongitudinalPhase[-]/1  "LongitudinalPhase[-]"
  __TDD__LongitudinalControl.LongitudinalPhase[-]/1 -> __TDO__LongitudinalControl/51  "LongitudinalPhase[-]"
  UserDefined1[-]___UNIQUE_1/1 -> __TDD__LongitudinalControl.UserDefined1[-]/1  "UserDefined1[-]"
  __TDD__LongitudinalControl.UserDefined1[-]/1 -> __TDO__LongitudinalControl/52  "UserDefined1[-]"
  UserDefined2[-]___UNIQUE_1/1 -> __TDD__LongitudinalControl.UserDefined2[-]/1  "UserDefined2[-]"
  __TDD__LongitudinalControl.UserDefined2[-]/1 -> __TDO__LongitudinalControl/53  "UserDefined2[-]"
  __TDO__LongitudinalControl/1 -> LongitudinalControl___UNIQUE_1/1  "LongitudinalControl"

== system SingleTrackCANoe/SimulationModel/VehicleControl/LongitudinalControl/ControlSystems/Longitudinal Controller/Acceleration Brake Input ==
  ControlInputs : Inport
  Action Port : ActionPort  InitializeStates=reset  PropagateVarSize=During execution  ActionPortLabel=case [ 1 ]:
  Bus Creator : BusCreator  Inputs=25  OutDataTypeStr=Bus: TD_BO_LongitudinalSpeedControlOutputs
      settings: InheritFromInputs=off
  Bus Selector3 : BusSelector  OutputSignals=AccPedalPos,BrakePedalPos,MainBrakePress,FrontLeftWheelBrakePress,FrontRightWheelBrakePress,RearLeftWheelBrakePress,RearRightWheelBrakePress,Rear2LeftWheelBrakePress,Rear2RightWheelBrakePress,Rear3LeftWheelBrakePress,Rear3RightWheelBrakePress,TrailerFrontLeftWheelBrakePress,TrailerFrontRightWheelBrakePress,TrailerRearLeftWheelBrakePress,TrailerRearRightWheelBrakePress,TrailerRear2LeftWheelBrakePress,TrailerRear2RightWheelBrakePress,TrailerRear3LeftWheelBrakePress,TrailerRear3RightWheelBrakePress
  Constant{,1..5} (6 alike) : Constant  Value=0
  Signal Conversion : SignalConversion  ConversionOutput=Nonvirtual bus  OverrideOpt=off
  ControlOutputs : Outport  VectorParamsAs1DForOutWhenUnconnected=off
  wires:
  Bus Selector3/19 -> Bus Creator/19  "<TrailerRear3RightWheelBrakePress>"
  Bus Selector3/16 -> Bus Creator/16  "<TrailerRear2LeftWheelBrakePress>"
  Bus Selector3/6 -> Bus Creator/6  "<RearLeftWheelBrakePress>"
  Bus Selector3/12 -> Bus Creator/12  "<TrailerFrontLeftWheelBrakePress>"
  Bus Selector3/15 -> Bus Creator/15  "<TrailerRearRightWheelBrakePress>"
  Bus Selector3/14 -> Bus Creator/14  "<TrailerRearLeftWheelBrakePress>"
  Bus Selector3/13 -> Bus Creator/13  "<TrailerFrontRightWheelBrakePress>"
  Bus Selector3/10 -> Bus Creator/10  "<Rear3LeftWheelBrakePress>"
  Bus Selector3/11 -> Bus Creator/11  "<Rear3RightWheelBrakePress>"
  Bus Selector3/17 -> Bus Creator/17  "<TrailerRear2RightWheelBrakePress>"
  Bus Selector3/5 -> Bus Creator/5  "<FrontRightWheelBrakePress>"
  Bus Selector3/7 -> Bus Creator/7  "<RearRightWheelBrakePress>"
  Bus Selector3/18 -> Bus Creator/18  "<TrailerRear3LeftWheelBrakePress>"
  Bus Selector3/4 -> Bus Creator/4  "<FrontLeftWheelBrakePress>"
  Bus Selector3/8 -> Bus Creator/8  "<Rear2LeftWheelBrakePress>"
  ControlInputs/1 -> Bus Selector3/1
  Bus Selector3/9 -> Bus Creator/9  "<Rear2RightWheelBrakePress>"
  Bus Selector3/1 -> Bus Creator/1  "<AccPedalPos>"
  Bus Selector3/2 -> Bus Creator/2  "<BrakePedalPos>"
  Bus Selector3/3 -> Bus Creator/3  "<MainBrakePress>"
  Constant/1 -> Bus Creator/20  "RefSpd"
  Constant1/1 -> Bus Creator/21  "RefSpdPreview"
  Constant2/1 -> Bus Creator/22  "RefSpdRestrospect"
  Constant3/1 -> Bus Creator/23  "RefAcc"
  Constant4/1 -> Bus Creator/24  "UserDefinedRefValue"
  Bus Creator/1 -> Signal Conversion/1
  Signal Conversion/1 -> ControlOutputs/1
  Constant5/1 -> Bus Creator/25  "BrakeSwitch"

== system SingleTrackCANoe/SimulationModel/VehicleControl/LongitudinalControl/ControlSystems/Longitudinal Controller/Acceleration Control ==
  ControlInputs : Inport
  CtrlSystemsAbscissae : Inport  Port=2
  VehicleInfo : Inport  Port=3
  Action Port : ActionPort  InitializeStates=reset  PropagateVarSize=During execution  ActionPortLabel=case [ 3 ]:
  "Acceleration Control " : LongitudinalControllerModules/Acceleration Control   SystemSampleTime=-1  VariantActivationTime=update diagram  Latency=0  AutoFrameSizeCalculation=off
  AccelerationControl : LongitudinalControllerModules/DataContainerAccelerationControl  DATA_NODE=MDL.VehicleControl.LongitudinalControl.ControlSystems.AccelerationControl  ProportionalGainAcc=MDL.VehicleControl.LongitudinalControl.ControlSystems.AccelerationControl.ProportionalGainAcc  IntegralGainAcc=MDL.VehicleControl.LongitudinalControl.ControlSystems.AccelerationControl.IntegralGainAcc  ProportionalGainDec=MDL.VehicleControl.LongitudinalControl.ControlSystems.AccelerationControl.ProportionalGainDec  IntegralGainDec=MDL.VehicleControl.LongitudinalControl.ControlSystems.AccelerationControl.IntegralGainDec  ProportionalGainConst=MDL.VehicleControl.LongitudinalControl.ControlSystems.AccelerationControl.ProportionalGainConst  IntegralGainConst=MDL.VehicleControl.LongitudinalControl.ControlSystems.AccelerationControl.IntegralGainConst  MinAcc=MDL.VehicleControl.LongitudinalControl.ControlSystems.AccelerationControl.MinAcc  MaxAcc=MDL.VehicleControl.LongitudinalControl.ControlSystems.AccelerationControl.MaxAcc
  Bus Selector : BusSelector  OutputSignals=Drivetrain_DrivetrainPhysics_EngSpd[rad/s]
  Bus Selector1 : BusSelector  OutputSignals=RefAcc
  ComputeBrakePedalPos : Subsystem
  ComputeIntEngTrq : Subsystem
  Feedforward Control : LongitudinalControllerModules/Feedforward Control  SystemSampleTime=-1  VariantActivationTime=update diagram  Latency=0  AutoFrameSizeCalculation=off
  Memory : Memory  InheritSampleTime=on
  Write To ControlOutputs : Subsystem
  ControlOutputs : Outport  VectorParamsAs1DForOutWhenUnconnected=off
  wires:
  ComputeBrakePedalPos/1(BrakePedalPos[0_1]) -> Write To ControlOutputs/1(BrakePedalPos[0_1])
  Memory/1 -> Write To ControlOutputs/4(RefAcc[rad/s])
  ComputeIntEngTrq/2(RefEngTrq[Nm]) -> Write To ControlOutputs/2(IntendedEngTrq[Nm])
  ComputeIntEngTrq/1(RefTireTrq[Nm]) -> ComputeBrakePedalPos/2(RefTireTrq[Nm])
  Bus Selector/1 -> Write To ControlOutputs/3(EngSpd[rad/s])  "<Drivetrain_DrivetrainPhysics_EngSpd[rad/s]>"
  "Acceleration Control "/1 -> ComputeIntEngTrq/3(ControlTrq[Nm])
  VehicleInfo/1 -> "Acceleration Control "/2, ComputeIntEngTrq/2(VehicleInfo), Bus Selector/1, Feedforward Control/2, ComputeBrakePedalPos/1(VehicleInfo)
  Feedforward Control/1 -> ComputeIntEngTrq/1(FeedforwardTrq[Nm])
  CtrlSystemsAbscissae/1 -> AccelerationControl/1
  ControlInputs/1 -> Bus Selector1/1
  AccelerationControl/1 -> "Acceleration Control "/1, Feedforward Control/1
  Bus Selector1/1 -> Feedforward Control/3, "Acceleration Control "/3, Memory/1  "<RefAcc>"
  Write To ControlOutputs/1(ControlOutputs) -> ControlOutputs/1

== system SingleTrackCANoe/SimulationModel/VehicleControl/LongitudinalControl/ControlSystems/Longitudinal Controller/Compute Acc Pedal Position ==
  note: TASK_LONG_ACC_BRAKE_INPUTS = 1;
      | 	TASK_LONG_SPEED_CONTROL = 2;
      | 	TASK_LONG_ACCELERATION_CONTROL = 3;
      | 	TASK_LONG_USER_DEFINED = 4;
  TaskIdentifier : Inport
  VehicleInfo : Inport  Port=2
  ControlOutputs : Inport  Port=3
  DelayEngTrq : LongitudinalControllerModules/DelayEngTrq  SystemSampleTime=-1  VariantActivationTime=update diagram  Latency=0  AutoFrameSizeCalculation=off
  Invert Acc Pedal : Subsystem
  Merge : Merge
  Pass Through ControlOutputs : Subsystem  TreatAsAtomicUnit=on
  Switch Case : SwitchCase  CaseConditions={[0, 2, 3, 4], 1}  ShowDefaultCase=off
  ModifiedControlOutputs : Outport  VectorParamsAs1DForOutWhenUnconnected=off
  wires:
  DelayEngTrq/1 -> Invert Acc Pedal/1(VehicleInfo)
  VehicleInfo/1 -> DelayEngTrq/1
  ControlOutputs/1 -> DelayEngTrq/2
  TaskIdentifier/1 -> Switch Case/1
  Switch Case/1 -> Invert Acc Pedal/Action
  Switch Case/2 -> Pass Through ControlOutputs/Action
  Invert Acc Pedal/1(ModifiedControlOutputs) -> Merge/1
  Pass Through ControlOutputs/1(ModifiedControlOutputs) -> Merge/2
  Merge/1 -> ModifiedControlOutputs/1
  DelayEngTrq/2 -> Invert Acc Pedal/2(ControlOutputs), Pass Through ControlOutputs/1(ControlOutputs)

== system SingleTrackCANoe/SimulationModel/VehicleControl/LongitudinalControl/ControlSystems/Longitudinal Controller/Initialization ==
  Action Port : ActionPort  InitializeStates=reset  PropagateVarSize=During execution  ActionPortLabel=case [ 0 ]:
  Initialize SpeedControlOutput Bus : Constant  Value=0  OutDataTypeStr=Bus: TD_BO_LongitudinalSpeedControlOutputs
  ControlOutputs : Outport  VectorParamsAs1DForOutWhenUnconnected=off
  wires:
  Initialize SpeedControlOutput Bus/1 -> ControlOutputs/1

== system SingleTrackCANoe/SimulationModel/VehicleControl/LongitudinalControl/ControlSystems/Longitudinal Controller/Speed Control ==
  ControlInputs : Inport
  SpeedControlParameters : Inport  Port=2
  VehicleInfo : Inport  Port=3
  Action Port : ActionPort  InitializeStates=reset  PropagateVarSize=During execution  ActionPortLabel=case [ 2 ]:
  Abs : Abs
  Bus Selector : BusSelector  OutputSignals=RefSpd,RefSpdPreview,RefSpdRetrospect,RefAcc
  Load Torque Vehicle : Subsystem
  Mux : Mux  Inputs=3
  Preprocessing VehicleInfo : Subsystem
  Product : Product  RndMeth=Zero
  SpeedController : LongitudinalControllerModules/SpeedControl  SystemSampleTime=-1  VariantActivationTime=update diagram  Latency=0  AutoFrameSizeCalculation=off
  Write to ControlOutputs : Subsystem
  ControlOutputs : Outport  VectorParamsAs1DForOutWhenUnconnected=off
  wires:
  SpeedController/5 -> Write to ControlOutputs/5(RefAcc[m/s**2])  "RefAcc"
  SpeedController/4 -> Write to ControlOutputs/4(RefSpd[m/s])  "RefSpd"
  Preprocessing VehicleInfo/8(FinalDriveRatio[-]) -> SpeedController/11
  Preprocessing VehicleInfo/7(MaxBrakeFrc[N]) -> Product/1, SpeedController/10
  Preprocessing VehicleInfo/4(DynamicTireRadius[m]) -> Load Torque Vehicle/2(TireRadius[m]), SpeedController/7
  SpeedController/3 -> Write to ControlOutputs/3(EngSpd[rad/s])  "EngSpd"
  Preprocessing VehicleInfo/9(LongAeroDragCoeff[-]) -> SpeedController/12
  SpeedController/2 -> Write to ControlOutputs/2(IntendedEngTrq[Nm])  "IntendedEngTrq"
  SpeedController/1 -> Write to ControlOutputs/1(AccPedalPos[0_1])  "AccPedalPos"
  Preprocessing VehicleInfo/18(SumMaxRollResistanceTrq[Nm]) -> Load Torque Vehicle/5(SumMaxRollResistanceTrq[Nm])
  Abs/1 -> SpeedController/1
  Preprocessing VehicleInfo/6(TractionCtrlFlag[0/1]) -> SpeedController/9
  Preprocessing VehicleInfo/11(ClutchPos[0_1]) -> SpeedController/14
  Bus Selector/2 -> Mux/2  "<RefSpdPreview>"
  Bus Selector/1 -> Mux/1  "<RefSpd>"
  Preprocessing VehicleInfo/19(VehMass[kg]) -> SpeedController/20, Load Torque Vehicle/6(VehMass [kg])
  Mux/1 -> Abs/1
  Preprocessing VehicleInfo/17(RoadSlopeLong[-]) -> Load Torque Vehicle/4(RoadSlopeLong [-])
  Product/1 -> Load Torque Vehicle/7(BrakeFrc[N])
  Bus Selector/3 -> Mux/3  "<RefSpdRetrospect>"
  SpeedController/6 -> Product/2, Write to ControlOutputs/6(BrakePedalPos[0_1])  "BrakePedalPos"
  Preprocessing VehicleInfo/16(AerodynamicFrc[N]) -> Load Torque Vehicle/3(AerodynamicFrc[N])
  Load Torque Vehicle/1(LoadTrq[Nm]) -> SpeedController/19
  Preprocessing VehicleInfo/2(EngSpd[rad/s]) -> SpeedController/5
  Preprocessing VehicleInfo/3(ExternalTrqs[Nm]) -> SpeedController/6
  ControlInputs/1 -> Bus Selector/1
  Preprocessing VehicleInfo/13(Gear[-4;20]) -> SpeedController/16
  Preprocessing VehicleInfo/1(VehSpd[m/s]) -> Load Torque Vehicle/1(VehSpd[m/s]), SpeedController/4
  Preprocessing VehicleInfo/5(VehAndWheelInrtl[kg*m**2]) -> SpeedController/8
  VehicleInfo/1 -> Preprocessing VehicleInfo/1(VehicleInfo)
  SpeedControlParameters/1 -> SpeedController/3
  Write to ControlOutputs/1(ControlOutputs) -> ControlOutputs/1
  Preprocessing VehicleInfo/10(AccPedalPos[0_1]) -> SpeedController/13
  Preprocessing VehicleInfo/12(EngInrtl[kg*m**2]) -> SpeedController/15
  Bus Selector/4 -> SpeedController/2  "<RefAcc>"
  Preprocessing VehicleInfo/14(FullAccPedalTrq[Nm]) -> SpeedController/17
  Preprocessing VehicleInfo/15(ZeroAccPedalTrq[Nm]) -> SpeedController/18

== system SingleTrackCANoe/SimulationModel/VehicleControl/LongitudinalControl/ControlSystems/Longitudinal Controller/User-defined Control ==
  ControlInputs : Inport
  VehicleInfo : Inport  Port=2
  SourceIdentifiers : Inport  Port=3
  Subtask Identifiers : Inport  Port=4
  Action Port : ActionPort  InitializeStates=reset  PropagateVarSize=During execution  ActionPortLabel=case [ 4 ]:
  UserDefinedControl : LongitudinalControllerModules/UserDefinedLongitudinalControl  DATA_NODE=MDL.VehicleControl.LongitudinalControl.ControlSystems.UserDefinedControl  ProportionalGain=MDL.VehicleControl.LongitudinalControl.ControlSystems.UserDefinedControl.SpdProportionalGain  IntegralGain=MDL.VehicleControl.LongitudinalControl.ControlSystems.UserDefinedControl.SpdIntegralGainTimeConst  DerivativeGain=MDL.VehicleControl.LongitudinalControl.ControlSystems.UserDefinedControl.SpdDerivativeGainTimeConst  DerivativeGainCompParam=MDL.VehicleControl.LongitudinalControl.ControlSystems.UserDefinedControl.SpdDerivativeGainEvalTimeConst  BrakePedalDelay=MDL.VehicleControl.LongitudinalControl.ControlSystems.UserDefinedControl.BrakePedalDelayConst  ControllerSpeedThres=MDL.VehicleControl.LongitudinalControl.ControlSystems.UserDefinedControl.ControllerSpdThres  BrakeProportionalGain=MDL.VehicleControl.LongitudinalControl.ControlSystems.UserDefinedControl.BrakeProportionalGain  BrakeIntegralGain=MDL.VehicleControl.LongitudinalControl.ControlSystems.UserDefinedControl.BrakeIntegralGain  BrakeDerivativeGain=MDL.VehicleControl.LongitudinalControl.ControlSystems.UserDefinedControl.BrakeDerivativeGain
  ControlOutputs : Outport  VectorParamsAs1DForOutWhenUnconnected=off
  wires:
  Subtask Identifiers/1 -> UserDefinedControl/1
  ControlInputs/1 -> UserDefinedControl/3
  VehicleInfo/1 -> UserDefinedControl/4
  SourceIdentifiers/1 -> UserDefinedControl/2
  UserDefinedControl/1 -> ControlOutputs/1

== system SingleTrackCANoe/SimulationModel/VehicleControl/LongitudinalControl/ControlSystemsPreprocessor/External Presetting of Controller /Presetting Source Identifiers ==
  note: SOURCE_NOMINALPATH = 1;
      | 	SOURCE_LANE = 2;
      | 	SOURCE_CONSTANT = 3;
      | 	SOURCE_TABLE_DISCRETE = 4;
      | 	SOURCE_TABLE_LINEAR = 5;
      | 	SOURCE_TABLE_CUBIC = 6;
      | 	SOURCE_TABLE_HAVERSINE = 7;
      | 	SOURCE_AUTOMATIC = 8;
      | 	SOURCE_SINE_TIME = 9;
      | 	SOURCE_SINE_PATH = 10;
      | 	SOURCE_HOLD = 11;
      | 	SOURCE_EXTERNAL = 12;
      | 	SOURCE_EXTERNAL_NOMINALPATH = 13;
      | 	SOURCE_EXTERNAL_LANE = 14;
  ExtCtrlVariablesEnforced : Inport
  SourceIdentifiers : Inport  Port=2
  Bus Selector : BusSelector  OutputSignals=CTRL_LongitudinalControl_RefSpdEnforced,CTRL_LongitudinalControl_RefAccEnforced,CTRL_LongitudinalControl_UserDefinedRefValueEnforced
  Bus Selector1 : BusSelector  OutputSignals=RefSpd,RefAcc,UserDefinedRefValue
  RefAccExternal : Constant  Value=vm_const('SOURCE_EXTERNAL')
  RefSpdExternal : Constant  Value=vm_const('SOURCE_EXTERNAL')
  SpeedCtrl_Spd : BusAssignment  AssignedSignals=RefSpd,RefSpdPreview,RefSpdRetrospect,RefAcc,UserDefinedRefValue
  Switch1 : Switch  Criteria=u2 > Threshold  OutDataTypeStr=Inherit: Inherit via back propagation
  Switch2 : Switch  Criteria=u2 > Threshold  OutDataTypeStr=Inherit: Inherit via back propagation
  Switch3 : Switch  Criteria=u2 > Threshold  OutDataTypeStr=Inherit: Inherit via back propagation
  UserDefinedRefValueExternal : Constant  Value=vm_const('SOURCE_EXTERNAL')
  ModifiedSourceIdentifiers : Outport  VectorParamsAs1DForOutWhenUnconnected=off
  wires:
  SpeedCtrl_Spd/1 -> ModifiedSourceIdentifiers/1
  Switch1/1 -> SpeedCtrl_Spd/2, SpeedCtrl_Spd/3, SpeedCtrl_Spd/4
  UserDefinedRefValueExternal/1 -> Switch2/1
  Bus Selector1/1 -> Switch1/3  "<RefSpd>"
  RefSpdExternal/1 -> Switch1/1
  SourceIdentifiers/1 -> Bus Selector1/1, SpeedCtrl_Spd/1
  ExtCtrlVariablesEnforced/1 -> Bus Selector/1
  Switch2/1 -> SpeedCtrl_Spd/6
  RefAccExternal/1 -> Switch3/1
  Switch3/1 -> SpeedCtrl_Spd/5
  Bus Selector1/2 -> Switch3/3  "<RefAcc>"
  Bus Selector1/3 -> Switch2/3  "<UserDefinedRefValue>"
  Bus Selector/2 -> Switch3/2  "<CTRL_LongitudinalControl_RefAccEnforced>"
  Bus Selector/1 -> Switch1/2  "<CTRL_LongitudinalControl_RefSpdEnforced>"
  Bus Selector/3 -> Switch2/2  "<CTRL_LongitudinalControl_UserDefinedRefValueEnforced>"

== system SingleTrackCANoe/SimulationModel/VehicleControl/LongitudinalControl/ControlSystemsPreprocessor/External Presetting of Controller /Presetting Task Identifiers ==
  note: TASK_LONG_ACC_BRAKE_INPUTS = 1;
      | 	TASK_LONG_SPEED_CONTROL = 2;
      | 	TASK_LONG_ACCELERATION_CONTROL = 3;
      | 	TASK_LONG_USER_DEFINED = 4;
  ExtCtrlVariablesEnforced : Inport
  TaskIdentifiers : Inport  Port=2
  Bus Creator : BusCreator  Inputs=2
  Bus Selector : BusSelector  OutputSignals=CTRL_LongitudinalControl_RefSpdEnforced,CTRL_LongitudinalControl_RefAccEnforced,CTRL_LongitudinalControl_UserDefinedRefValueEnforced  OutputAsBus=on
  Bus Selector1 : BusSelector  OutputSignals=Task[-],Subtask[-]
  Bus to Vector : BusToVector
  Demux : Demux  Outputs=2
  Gain : Gain  Gain=[3 2 1]
  MinMax : MinMax  Function=max
  Multiport Switch : MultiPortSwitch  DataPortOrder=Zero-based contiguous  Inputs=4  zeroidx=on
  Mux : Mux  Inputs=2
  Speed Control : Constant  Value=[vm_const('TASK_LONG_SPEED_CONTROL') 0]
  Speed Control1 : Constant  Value=[vm_const('TASK_LONG_ACCELERATION_CONTROL') 0]
  Speed Control2 : Constant  Value=[vm_const('TASK_LONG_USER_DEFINED') 0]
  ModifiedTaskIdentifiers : Outport  VectorParamsAs1DForOutWhenUnconnected=off
  wires:
  Mux/1 -> Multiport Switch/2
  MinMax/1 -> Multiport Switch/1
  Bus Selector/1 -> Bus to Vector/1
  Bus to Vector/1 -> Gain/1
  Gain/1 -> MinMax/1
  Bus Selector1/2 -> Mux/2  "<Subtask[-]>"
  Bus Selector1/1 -> Mux/1  "<Task[-]>"
  TaskIdentifiers/1 -> Bus Selector1/1
  Multiport Switch/1 -> Demux/1
  Demux/1 -> Bus Creator/1  "Task"
  Demux/2 -> Bus Creator/2  "Subtask"
  ExtCtrlVariablesEnforced/1 -> Bus Selector/1
  Bus Creator/1 -> ModifiedTaskIdentifiers/1
  Speed Control/1 -> Multiport Switch/5
  Speed Control2/1 -> Multiport Switch/3
  Speed Control1/1 -> Multiport Switch/4

== system SingleTrackCANoe/SimulationModel/VehicleControl/LongitudinalControl/ControlSystemsPreprocessor/Generation of Hold Data/DefaultAction Subsystem ==
  HoldData : Inport
  Action Port : ActionPort  InitializeStates=reset  ActionPortLabel=default:
  HoldLongitudinalControlInputs : Outport  VectorParamsAs1DForOutWhenUnconnected=off
  wires:
  HoldData/1 -> HoldLongitudinalControlInputs/1
